simulink model "quadruped_2016"  (R2016a)
settings: Solver=ode23t  SolverMode=SingleTasking  StartTime=0.0  StopTime=8  RelTol=1e-3
values from neighbouring files (symbols this model uses):
  robot = Robot    [quadruped_sim_param.m]
undefined symbols (not defined in the file or in its folder): sigbuilder_block, X, Y, Z
undefined symbols (not defined in the file): plane
libraries: sm_lib x138, nesl_utility x66, simulink x24, Contact_Forces_Lib x12
(part 2 of 5)

== system quadruped_2016/robot/FR/hip ==
  pos : Inport
  Rigid Transform1 : sm_lib/Frames and Transforms/Rigid Transform  TranslationMethod=StandardAxis  TranslationStandardOffset=Hip.gearboxCorrection  TranslationLengthUnit=mm  TranslationStandardAxis=-Z  TranslationCartesianOffset=50  TranslationROffset=0  TranslationROffsetUnits=m  TranslationZOffset=0  TranslationZOffsetUnits=m  TranslationThetaOffset=0  TranslationThetaOffsetUnits=deg  RotationMethod=None  RotationAngleUnits=deg  RotationStandardAxis=-X  RotationAngle=180  RotationArbitraryAxis=[0 0 1]  FollAlignAxisA=+X  BaseAlignAxisA=+Y  FollAlignAxisB=+Y  BaseAlignAxisB=+Z  RotationSequenceAxes=FollowerAxes  RotationSequence=XYZ  RotationSequenceAngles=[180 0 180]  RotationSequenceAnglesUnits=deg  RotationMatrix=[1 0 0; 0 1 0; 0 0 1]
  Rigid Transform6 : sm_lib/Frames and Transforms/Rigid Transform  TranslationMethod=Cartesian  TranslationStandardOffset=0.3  TranslationLengthUnit=mm  TranslationStandardAxis=+X  TranslationCartesianOffset=Hip.legGbxOft  TranslationROffset=0  TranslationROffsetUnits=m  TranslationZOffset=0  TranslationZOffsetUnits=m  TranslationThetaOffset=0  TranslationThetaOffsetUnits=deg  RotationMethod=StandardAxis  RotationAngleUnits=deg  RotationStandardAxis=-X  RotationAngle=90  RotationArbitraryAxis=[0 0 1]  FollAlignAxisA=+X  BaseAlignAxisA=+Y  FollAlignAxisB=+Y  BaseAlignAxisB=+Z  RotationSequenceAxes=FollowerAxes  RotationSequence=XYX  RotationSequenceAngles=[0 0 0]  RotationSequenceAnglesUnits=deg  RotationMatrix=[1 0 0; 0 1 0; 0 0 1]
  Rigid Transform7 : sm_lib/Frames and Transforms/Rigid Transform  TranslationMethod=Cartesian  TranslationStandardOffset=0.3  TranslationLengthUnit=mm  TranslationStandardAxis=+X  TranslationCartesianOffset=Hip.legOft  TranslationROffset=0  TranslationROffsetUnits=m  TranslationZOffset=0  TranslationZOffsetUnits=m  TranslationThetaOffset=0  TranslationThetaOffsetUnits=deg  RotationMethod=RotationSequence  RotationAngleUnits=deg  RotationStandardAxis=-X  RotationAngle=180  RotationArbitraryAxis=[0 0 1]  FollAlignAxisA=+X  BaseAlignAxisA=+Y  FollAlignAxisB=+Y  BaseAlignAxisB=+Z  RotationSequenceAxes=FollowerAxes  RotationSequence=XYZ  RotationSequenceAngles=[0 0 180]  RotationSequenceAnglesUnits=deg  RotationMatrix=[1 0 0; 0 1 0; 0 0 1]
  Rigid Transform8 : sm_lib/Frames and Transforms/Rigid Transform  TranslationMethod=Cartesian  TranslationStandardOffset=0.3  TranslationLengthUnit=mm  TranslationStandardAxis=+X  TranslationCartesianOffset=Hip.kneeGbxOft  TranslationROffset=0  TranslationROffsetUnits=m  TranslationZOffset=0  TranslationZOffsetUnits=m  TranslationThetaOffset=0  TranslationThetaOffsetUnits=deg  RotationMethod=StandardAxis  RotationAngleUnits=deg  RotationStandardAxis=-X  RotationAngle=90  RotationArbitraryAxis=[0 0 1]  FollAlignAxisA=+X  BaseAlignAxisA=+Y  FollAlignAxisB=+Y  BaseAlignAxisB=+Z  RotationSequenceAxes=FollowerAxes  RotationSequence=XYX  RotationSequenceAngles=[0 0 0]  RotationSequenceAnglesUnits=deg  RotationMatrix=[1 0 0; 0 1 0; 0 0 1]
  Sphere to Plane Force1 : Contact_Forces_Lib/3D/Sphere to Plane Force  sphere_rad=Leg.lower_joint.sphere_rad  plane_lenx=plane_dim(1)  plane_leny=plane_dim(2)  plane_depth=plane_dim(3)/2  force_law=Linear  k_contact=1e4  b_contact=1e2  pen_full_damp_F=1e-4  pen_exponent=1  custom_param_1=1  custom_param_2=1  friction_law=Stick-Slip Continuous  mu_kinetic=Leg.lower_joint.kine_frict  mu_static=Leg.lower_joint.stat_frict  v_thr=0.001  vis_on=off  vis_opc_en=0  vis_len_plaBz=0.005  vis_clr=[0.9 0.2 0.2]  vis_opc=0.7
  Terminator : Terminator
  hip motor : sm_lib/Body Elements/Solid  GraphicAmbientColor=[0.15 0.15 0.15 1.0]  BasedOnType=Mass  CenterOfMass=[0 0 0]  CenterOfMassUnits=m  GraphicDiffuseColor=Hip.GbxColor  CylinderLength=Hip.gearboxThickness  CylinderLengthUnits=mm  CylinderRadius=Hip.gearboxRadius  CylinderRadiusUnits=mm  Density=1000  DensityUnits=kg/m^3  DoExposeReferenceFrame=on  GraphicEmissiveColor=[0.0 0.0 0.0 1.0]  ExportEntireGeometry=off  SerializedFrames=<Frames/>  MarkerShape=Sphere  MarkerSize=10  GraphicType=FromGeometry  InertiaType=CalculateFromGeometry  Mass=Hip.gearboxMass  MassUnits=g  MomentsOfInertia=[1 1 1]  MomentsOfInertiaUnits=kg*m^2  GraphicOpacity=1.0  ProductsOfInertia=[0 0 0]  ProductsOfInertiaUnits=kg*m^2  GraphicShininess=75  GraphicSpecularColor=[0.5 0.5 0.5 1.0]  GraphicVisPropType=SimpleVisualProperties  GeometryShape=Cylinder
  joint : Subsystem  mask{Joint=Hip.joint}
  knee motor : sm_lib/Body Elements/Solid  GraphicAmbientColor=[0.15 0.15 0.15 1.0]  BasedOnType=Mass  CenterOfMass=[0 0 0]  CenterOfMassUnits=m  GraphicDiffuseColor=Hip.GbxColor  CylinderLength=Hip.gearboxThickness  CylinderLengthUnits=mm  CylinderRadius=Hip.gearboxRadius  CylinderRadiusUnits=mm  Density=1000  DensityUnits=kg/m^3  DoExposeReferenceFrame=on  GraphicEmissiveColor=[0.0 0.0 0.0 1.0]  ExportEntireGeometry=off  SerializedFrames=<Frames/>  MarkerShape=Sphere  MarkerSize=10  GraphicType=FromGeometry  InertiaType=CalculateFromGeometry  Mass=Hip.gearboxMass  MassUnits=g  MomentsOfInertia=[1 1 1]  MomentsOfInertiaUnits=kg*m^2  GraphicOpacity=1.0  ProductsOfInertia=[0 0 0]  ProductsOfInertiaUnits=kg*m^2  GraphicShininess=75  GraphicSpecularColor=[0.5 0.5 0.5 1.0]  GraphicVisPropType=SimpleVisualProperties  GeometryShape=Cylinder
  leg motor : sm_lib/Body Elements/Solid  GraphicAmbientColor=[0.15 0.15 0.15 1.0]  BasedOnType=Mass  CenterOfMass=[0 0 0]  CenterOfMassUnits=m  GraphicDiffuseColor=Hip.GbxColor  CylinderLength=Hip.gearboxThickness  CylinderLengthUnits=mm  CylinderRadius=Hip.gearboxRadius  CylinderRadiusUnits=mm  Density=1000  DensityUnits=kg/m^3  DoExposeReferenceFrame=on  GraphicEmissiveColor=[0.0 0.0 0.0 1.0]  ExportEntireGeometry=off  SerializedFrames=<Frames/>  MarkerShape=Sphere  MarkerSize=10  GraphicType=FromGeometry  InertiaType=CalculateFromGeometry  Mass=Hip.gearboxMass  MassUnits=g  MomentsOfInertia=[1 1 1]  MomentsOfInertiaUnits=kg*m^2  GraphicOpacity=1.0  ProductsOfInertia=[0 0 0]  ProductsOfInertiaUnits=kg*m^2  GraphicShininess=75  GraphicSpecularColor=[0.5 0.5 0.5 1.0]  GraphicVisPropType=SimpleVisualProperties  GeometryShape=Cylinder
  B : PMIOPort  Side=Left
  F : PMIOPort  Port=2  Side=Right
  plane : PMIOPort  Port=3  Side=Right
  p : Outport
  wires:
  Sphere to Plane Force1/1 -> Terminator/1
  pos/1 -> joint/1(in)
  joint/1(p) -> p/1
  connections:
  Rigid Transform7/RConn1 -- F/RConn1
  Rigid Transform6/RConn1 -- leg motor/RConn1 -- Rigid Transform7/LConn1
  Rigid Transform8/RConn1 -- knee motor/RConn1 -- Sphere to Plane Force1/LConn1
  Sphere to Plane Force1/RConn1 -- plane/RConn1
  B/RConn1 -- Rigid Transform1/LConn1
  joint/RConn1 -- Rigid Transform6/LConn1 -- Rigid Transform8/LConn1 -- hip motor/RConn1
  Rigid Transform1/RConn1 -- joint/LConn1

== system quadruped_2016/robot/FR/leg ==
  up pos : Inport
  lo pos : Inport  Port=2
  Bus Creator : BusCreator  Inputs=2
  Sphere to Plane Force1 : Contact_Forces_Lib/3D/Sphere to Plane Force  sphere_rad=Leg.lower_joint.sphere_rad  plane_lenx=plane_dim(1)  plane_leny=plane_dim(2)  plane_depth=plane_dim(3)/2  force_law=Linear  k_contact=1e4  b_contact=1e2  pen_full_damp_F=1e-4  pen_exponent=1  custom_param_1=1  custom_param_2=1  friction_law=Stick-Slip Continuous  mu_kinetic=Leg.lower_joint.kine_frict  mu_static=Leg.lower_joint.stat_frict  v_thr=0.001  vis_on=off  vis_opc_en=0  vis_len_plaBz=0.005  vis_clr=[0.9 0.2 0.2]  vis_opc=0.7
  Sphere to Plane Force2 : Contact_Forces_Lib/3D/Sphere to Plane Force  sphere_rad=Leg.lower_joint.sphere_rad  plane_lenx=plane_dim(1)  plane_leny=plane_dim(2)  plane_depth=plane_dim(3)/2  force_law=Linear  k_contact=1e4  b_contact=1e2  pen_full_damp_F=1e-4  pen_exponent=1  custom_param_1=1  custom_param_2=1  friction_law=Stick-Slip Continuous  mu_kinetic=Leg.lower_joint.kine_frict  mu_static=Leg.lower_joint.stat_frict  v_thr=0.001  vis_on=off  vis_opc_en=0  vis_len_plaBz=0.005  vis_clr=[0.9 0.2 0.2]  vis_opc=0.7
  Terminator : Terminator
  Terminator1 : Terminator
  Top2 : sm_lib/Frames and Transforms/Rigid Transform  TranslationMethod=StandardAxis  TranslationStandardOffset=Leg.lower_joint.sphere_rad  TranslationLengthUnit=m  TranslationStandardAxis=+X  TranslationCartesianOffset=[0 0 0.1]  TranslationROffset=0  TranslationROffsetUnits=m  TranslationZOffset=0  TranslationZOffsetUnits=m  TranslationThetaOffset=0  TranslationThetaOffsetUnits=deg  RotationMethod=None  RotationAngleUnits=deg  RotationStandardAxis=+Y  RotationAngle=90  RotationArbitraryAxis=[0 0 1]  FollAlignAxisA=+X  BaseAlignAxisA=+Y  FollAlignAxisB=+Y  BaseAlignAxisB=+Z  RotationSequenceAxes=FollowerAxes  RotationSequence=XYX  RotationSequenceAngles=[0 0 0]  RotationSequenceAnglesUnits=deg  RotationMatrix=[1 0 0; 0 1 0; 0 0 1]
  lower joint : Subsystem  mask{Leg_joint=Leg.lower_joint}
  upper joint : Subsystem  mask{Leg_joint=Leg.upper_joint}
  B : PMIOPort  Side=Left
  plane : PMIOPort  Port=2  Side=Right
  p : Outport
  wires:
  Sphere to Plane Force2/1 -> Terminator/1
  Sphere to Plane Force1/1 -> Terminator1/1
  up pos/1 -> upper joint/1(pos)
  lo pos/1 -> lower joint/1(pos)
  Bus Creator/1 -> p/1
  lower joint/1(p) -> Bus Creator/1  "lower joint data"
  upper joint/1(p) -> Bus Creator/2  "upper jount data"
  connections:
  Sphere to Plane Force2/LConn1 -- upper joint/RConn1 -- lower joint/LConn1
  upper joint/LConn1 -- B/RConn1
  Top2/LConn1 -- Sphere to Plane Force1/LConn1
  plane/RConn1 -- Sphere to Plane Force1/RConn1 -- Sphere to Plane Force2/RConn1
  lower joint/RConn1 -- Top2/RConn1

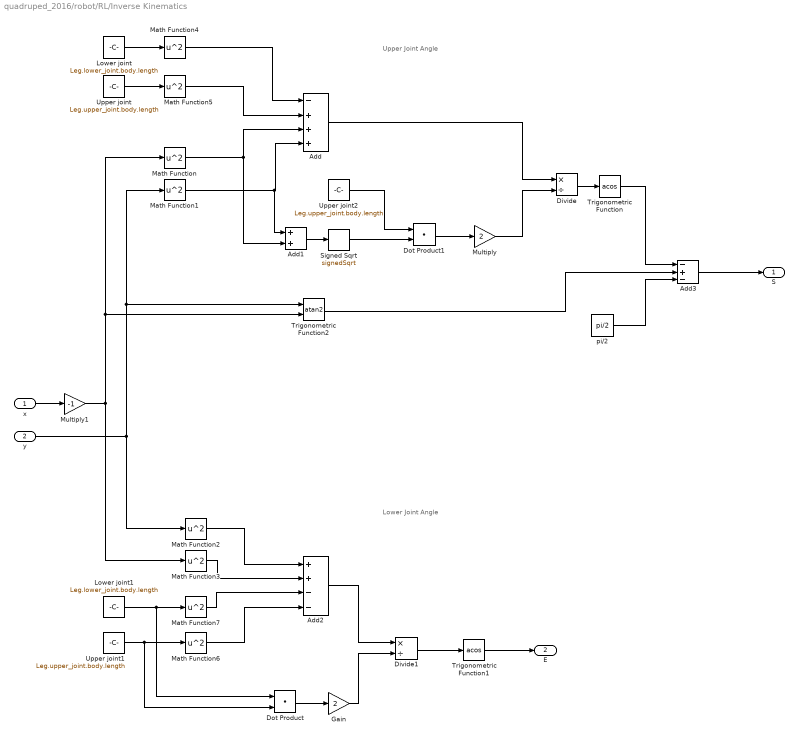
== system quadruped_2016/robot/RL/Inverse Kinematics  ==
  note: Upper Joint Angle
  note: Lower Joint Angle
  x : Inport
  y : Inport  Port=2
  Add : Sum  Inputs=-+++
  Add1 : Sum
  Add2 : Sum  Inputs=++--
  Add3 : Sum  Inputs=-+-
  Divide : Product  Inputs=*/
  Divide1 : Product  Inputs=*/
  Dot Product : DotProduct  InputSameDT=on  OutDataTypeStr=Inherit: Inherit via internal rule
  Dot Product1 : DotProduct  InputSameDT=on  OutDataTypeStr=Inherit: Inherit via internal rule
  Gain : Gain  Gain=2
  Lower joint : Constant  Value=Leg.lower_joint.body.length
  Lower joint1 : Constant  Value=Leg.lower_joint.body.length
  Math Function{,1..7} (8 alike) : Math  Operator=square  SaturateOnIntegerOverflow=on
  Multiply : Gain  Gain=2
  Multiply1 : Gain  Gain=-1
  Signed Sqrt : Sqrt  Operator=signedSqrt  SaturateOnIntegerOverflow=on
  Trigonometric Function : Trigonometry  Operator=acos
  Trigonometric Function1 : Trigonometry  Operator=acos
  Trigonometric Function2 : Trigonometry  Operator=atan2
  Upper joint : Constant  Value=Leg.upper_joint.body.length
  Upper joint1 : Constant  Value=Leg.upper_joint.body.length
  Upper joint2 : Constant  Value=Leg.upper_joint.body.length
  pi/2 : Constant  Value=pi/2
  S : Outport
  E : Outport  Port=2
  wires:
  y/1 -> Trigonometric Function2/1, Math Function1/1, Math Function2/1
  Lower joint/1 -> Math Function4/1
  Upper joint/1 -> Math Function5/1
  Math Function/1 -> Add1/2, Add/3
  Math Function1/1 -> Add1/1, Add/4
  Add1/1 -> Signed Sqrt/1
  Add/1 -> Divide/1
  Divide1/1 -> Trigonometric Function1/1
  Dot Product/1 -> Gain/1
  Add2/1 -> Divide1/1
  Gain/1 -> Divide1/2
  Divide/1 -> Trigonometric Function/1
  Trigonometric Function1/1 -> E/1
  Math Function2/1 -> Add2/1
  Math Function3/1 -> Add2/2
  Lower joint1/1 -> Math Function7/1, Dot Product/1
  Upper joint1/1 -> Dot Product/2, Math Function6/1
  Trigonometric Function/1 -> Add3/1
  Trigonometric Function2/1 -> Add3/2
  Add3/1 -> S/1
  Math Function5/1 -> Add/2
  Math Function4/1 -> Add/1
  Math Function7/1 -> Add2/3
  Math Function6/1 -> Add2/4
  Multiply/1 -> Divide/2
  Dot Product1/1 -> Multiply/1
  Signed Sqrt/1 -> Dot Product1/2
  Upper joint2/1 -> Dot Product1/1
  pi/2/1 -> Add3/3
  x/1 -> Multiply1/1
  Multiply1/1 -> Trigonometric Function2/2, Math Function/1, Math Function3/1

== system quadruped_2016/robot/RL/hip ==
  pos : Inport
  Rigid Transform1 : sm_lib/Frames and Transforms/Rigid Transform  TranslationMethod=StandardAxis  TranslationStandardOffset=Hip.gearboxCorrection  TranslationLengthUnit=mm  TranslationStandardAxis=-Z  TranslationCartesianOffset=50  TranslationROffset=0  TranslationROffsetUnits=m  TranslationZOffset=0  TranslationZOffsetUnits=m  TranslationThetaOffset=0  TranslationThetaOffsetUnits=deg  RotationMethod=None  RotationAngleUnits=deg  RotationStandardAxis=-X  RotationAngle=180  RotationArbitraryAxis=[0 0 1]  FollAlignAxisA=+X  BaseAlignAxisA=+Y  FollAlignAxisB=+Y  BaseAlignAxisB=+Z  RotationSequenceAxes=FollowerAxes  RotationSequence=XYZ  RotationSequenceAngles=[180 0 180]  RotationSequenceAnglesUnits=deg  RotationMatrix=[1 0 0; 0 1 0; 0 0 1]
  Rigid Transform6 : sm_lib/Frames and Transforms/Rigid Transform  TranslationMethod=Cartesian  TranslationStandardOffset=0.3  TranslationLengthUnit=mm  TranslationStandardAxis=+X  TranslationCartesianOffset=Hip.legGbxOft  TranslationROffset=0  TranslationROffsetUnits=m  TranslationZOffset=0  TranslationZOffsetUnits=m  TranslationThetaOffset=0  TranslationThetaOffsetUnits=deg  RotationMethod=StandardAxis  RotationAngleUnits=deg  RotationStandardAxis=-X  RotationAngle=90  RotationArbitraryAxis=[0 0 1]  FollAlignAxisA=+X  BaseAlignAxisA=+Y  FollAlignAxisB=+Y  BaseAlignAxisB=+Z  RotationSequenceAxes=FollowerAxes  RotationSequence=XYX  RotationSequenceAngles=[0 0 0]  RotationSequenceAnglesUnits=deg  RotationMatrix=[1 0 0; 0 1 0; 0 0 1]
  Rigid Transform7 : sm_lib/Frames and Transforms/Rigid Transform  TranslationMethod=Cartesian  TranslationStandardOffset=0.3  TranslationLengthUnit=mm  TranslationStandardAxis=+X  TranslationCartesianOffset=Hip.legOft  TranslationROffset=0  TranslationROffsetUnits=m  TranslationZOffset=0  TranslationZOffsetUnits=m  TranslationThetaOffset=0  TranslationThetaOffsetUnits=deg  RotationMethod=RotationSequence  RotationAngleUnits=deg  RotationStandardAxis=-X  RotationAngle=180  RotationArbitraryAxis=[0 0 1]  FollAlignAxisA=+X  BaseAlignAxisA=+Y  FollAlignAxisB=+Y  BaseAlignAxisB=+Z  RotationSequenceAxes=FollowerAxes  RotationSequence=XYZ  RotationSequenceAngles=[0 0 180]  RotationSequenceAnglesUnits=deg  RotationMatrix=[1 0 0; 0 1 0; 0 0 1]
  Rigid Transform8 : sm_lib/Frames and Transforms/Rigid Transform  TranslationMethod=Cartesian  TranslationStandardOffset=0.3  TranslationLengthUnit=mm  TranslationStandardAxis=+X  TranslationCartesianOffset=Hip.kneeGbxOft  TranslationROffset=0  TranslationROffsetUnits=m  TranslationZOffset=0  TranslationZOffsetUnits=m  TranslationThetaOffset=0  TranslationThetaOffsetUnits=deg  RotationMethod=StandardAxis  RotationAngleUnits=deg  RotationStandardAxis=-X  RotationAngle=90  RotationArbitraryAxis=[0 0 1]  FollAlignAxisA=+X  BaseAlignAxisA=+Y  FollAlignAxisB=+Y  BaseAlignAxisB=+Z  RotationSequenceAxes=FollowerAxes  RotationSequence=XYX  RotationSequenceAngles=[0 0 0]  RotationSequenceAnglesUnits=deg  RotationMatrix=[1 0 0; 0 1 0; 0 0 1]
  Sphere to Plane Force1 : Contact_Forces_Lib/3D/Sphere to Plane Force  sphere_rad=Leg.lower_joint.sphere_rad  plane_lenx=plane_dim(1)  plane_leny=plane_dim(2)  plane_depth=plane_dim(3)/2  force_law=Linear  k_contact=1e4  b_contact=1e2  pen_full_damp_F=1e-4  pen_exponent=1  custom_param_1=1  custom_param_2=1  friction_law=Stick-Slip Continuous  mu_kinetic=Leg.lower_joint.kine_frict  mu_static=Leg.lower_joint.stat_frict  v_thr=0.001  vis_on=off  vis_opc_en=0  vis_len_plaBz=0.005  vis_clr=[0.9 0.2 0.2]  vis_opc=0.7
  Terminator : Terminator
  hip motor : sm_lib/Body Elements/Solid  GraphicAmbientColor=[0.15 0.15 0.15 1.0]  BasedOnType=Mass  CenterOfMass=[0 0 0]  CenterOfMassUnits=m  GraphicDiffuseColor=Hip.GbxColor  CylinderLength=Hip.gearboxThickness  CylinderLengthUnits=mm  CylinderRadius=Hip.gearboxRadius  CylinderRadiusUnits=mm  Density=1000  DensityUnits=kg/m^3  DoExposeReferenceFrame=on  GraphicEmissiveColor=[0.0 0.0 0.0 1.0]  ExportEntireGeometry=off  SerializedFrames=<Frames/>  MarkerShape=Sphere  MarkerSize=10  GraphicType=FromGeometry  InertiaType=CalculateFromGeometry  Mass=Hip.gearboxMass  MassUnits=g  MomentsOfInertia=[1 1 1]  MomentsOfInertiaUnits=kg*m^2  GraphicOpacity=1.0  ProductsOfInertia=[0 0 0]  ProductsOfInertiaUnits=kg*m^2  GraphicShininess=75  GraphicSpecularColor=[0.5 0.5 0.5 1.0]  GraphicVisPropType=SimpleVisualProperties  GeometryShape=Cylinder
  joint : Subsystem  mask{Joint=Hip.joint}
  knee motor : sm_lib/Body Elements/Solid  GraphicAmbientColor=[0.15 0.15 0.15 1.0]  BasedOnType=Mass  CenterOfMass=[0 0 0]  CenterOfMassUnits=m  GraphicDiffuseColor=Hip.GbxColor  CylinderLength=Hip.gearboxThickness  CylinderLengthUnits=mm  CylinderRadius=Hip.gearboxRadius  CylinderRadiusUnits=mm  Density=1000  DensityUnits=kg/m^3  DoExposeReferenceFrame=on  GraphicEmissiveColor=[0.0 0.0 0.0 1.0]  ExportEntireGeometry=off  SerializedFrames=<Frames/>  MarkerShape=Sphere  MarkerSize=10  GraphicType=FromGeometry  InertiaType=CalculateFromGeometry  Mass=Hip.gearboxMass  MassUnits=g  MomentsOfInertia=[1 1 1]  MomentsOfInertiaUnits=kg*m^2  GraphicOpacity=1.0  ProductsOfInertia=[0 0 0]  ProductsOfInertiaUnits=kg*m^2  GraphicShininess=75  GraphicSpecularColor=[0.5 0.5 0.5 1.0]  GraphicVisPropType=SimpleVisualProperties  GeometryShape=Cylinder
  leg motor : sm_lib/Body Elements/Solid  GraphicAmbientColor=[0.15 0.15 0.15 1.0]  BasedOnType=Mass  CenterOfMass=[0 0 0]  CenterOfMassUnits=m  GraphicDiffuseColor=Hip.GbxColor  CylinderLength=Hip.gearboxThickness  CylinderLengthUnits=mm  CylinderRadius=Hip.gearboxRadius  CylinderRadiusUnits=mm  Density=1000  DensityUnits=kg/m^3  DoExposeReferenceFrame=on  GraphicEmissiveColor=[0.0 0.0 0.0 1.0]  ExportEntireGeometry=off  SerializedFrames=<Frames/>  MarkerShape=Sphere  MarkerSize=10  GraphicType=FromGeometry  InertiaType=CalculateFromGeometry  Mass=Hip.gearboxMass  MassUnits=g  MomentsOfInertia=[1 1 1]  MomentsOfInertiaUnits=kg*m^2  GraphicOpacity=1.0  ProductsOfInertia=[0 0 0]  ProductsOfInertiaUnits=kg*m^2  GraphicShininess=75  GraphicSpecularColor=[0.5 0.5 0.5 1.0]  GraphicVisPropType=SimpleVisualProperties  GeometryShape=Cylinder
  B : PMIOPort  Side=Left
  F : PMIOPort  Port=2  Side=Right
  plane : PMIOPort  Port=3  Side=Right
  p : Outport
  wires:
  Sphere to Plane Force1/1 -> Terminator/1
  pos/1 -> joint/1(in)
  joint/1(p) -> p/1
  connections:
  Rigid Transform7/RConn1 -- F/RConn1
  Rigid Transform6/RConn1 -- leg motor/RConn1 -- Rigid Transform7/LConn1
  Rigid Transform8/RConn1 -- knee motor/RConn1 -- Sphere to Plane Force1/LConn1
  Sphere to Plane Force1/RConn1 -- plane/RConn1
  B/RConn1 -- Rigid Transform1/LConn1
  joint/RConn1 -- Rigid Transform6/LConn1 -- Rigid Transform8/LConn1 -- hip motor/RConn1
  Rigid Transform1/RConn1 -- joint/LConn1

== system quadruped_2016/robot/RL/leg ==
  up pos : Inport
  lo pos : Inport  Port=2
  Bus Creator : BusCreator  Inputs=2
  Sphere to Plane Force1 : Contact_Forces_Lib/3D/Sphere to Plane Force  sphere_rad=Leg.lower_joint.sphere_rad  plane_lenx=plane_dim(1)  plane_leny=plane_dim(2)  plane_depth=plane_dim(3)/2  force_law=Linear  k_contact=1e4  b_contact=1e2  pen_full_damp_F=1e-4  pen_exponent=1  custom_param_1=1  custom_param_2=1  friction_law=Stick-Slip Continuous  mu_kinetic=Leg.lower_joint.kine_frict  mu_static=Leg.lower_joint.stat_frict  v_thr=0.001  vis_on=off  vis_opc_en=0  vis_len_plaBz=0.005  vis_clr=[0.9 0.2 0.2]  vis_opc=0.7
  Sphere to Plane Force2 : Contact_Forces_Lib/3D/Sphere to Plane Force  sphere_rad=Leg.lower_joint.sphere_rad  plane_lenx=plane_dim(1)  plane_leny=plane_dim(2)  plane_depth=plane_dim(3)/2  force_law=Linear  k_contact=1e4  b_contact=1e2  pen_full_damp_F=1e-4  pen_exponent=1  custom_param_1=1  custom_param_2=1  friction_law=Stick-Slip Continuous  mu_kinetic=Leg.lower_joint.kine_frict  mu_static=Leg.lower_joint.stat_frict  v_thr=0.001  vis_on=off  vis_opc_en=0  vis_len_plaBz=0.005  vis_clr=[0.9 0.2 0.2]  vis_opc=0.7
  Terminator : Terminator
  Terminator1 : Terminator
  Top2 : sm_lib/Frames and Transforms/Rigid Transform  TranslationMethod=StandardAxis  TranslationStandardOffset=Leg.lower_joint.sphere_rad  TranslationLengthUnit=m  TranslationStandardAxis=+X  TranslationCartesianOffset=[0 0 0.1]  TranslationROffset=0  TranslationROffsetUnits=m  TranslationZOffset=0  TranslationZOffsetUnits=m  TranslationThetaOffset=0  TranslationThetaOffsetUnits=deg  RotationMethod=None  RotationAngleUnits=deg  RotationStandardAxis=+Y  RotationAngle=90  RotationArbitraryAxis=[0 0 1]  FollAlignAxisA=+X  BaseAlignAxisA=+Y  FollAlignAxisB=+Y  BaseAlignAxisB=+Z  RotationSequenceAxes=FollowerAxes  RotationSequence=XYX  RotationSequenceAngles=[0 0 0]  RotationSequenceAnglesUnits=deg  RotationMatrix=[1 0 0; 0 1 0; 0 0 1]
  lower joint : Subsystem  mask{Leg_joint=Leg.lower_joint}
  upper joint : Subsystem  mask{Leg_joint=Leg.upper_joint}
  B : PMIOPort  Side=Left
  plane : PMIOPort  Port=2  Side=Right
  p : Outport
  wires:
  Sphere to Plane Force2/1 -> Terminator/1
  Sphere to Plane Force1/1 -> Terminator1/1
  up pos/1 -> upper joint/1(pos)
  lo pos/1 -> lower joint/1(pos)
  Bus Creator/1 -> p/1
  lower joint/1(p) -> Bus Creator/1  "lower joint data"
  upper joint/1(p) -> Bus Creator/2  "upper jount data"
  connections:
  Sphere to Plane Force2/LConn1 -- upper joint/RConn1 -- lower joint/LConn1
  upper joint/LConn1 -- B/RConn1
  Top2/LConn1 -- Sphere to Plane Force1/LConn1
  plane/RConn1 -- Sphere to Plane Force1/RConn1 -- Sphere to Plane Force2/RConn1
  lower joint/RConn1 -- Top2/RConn1

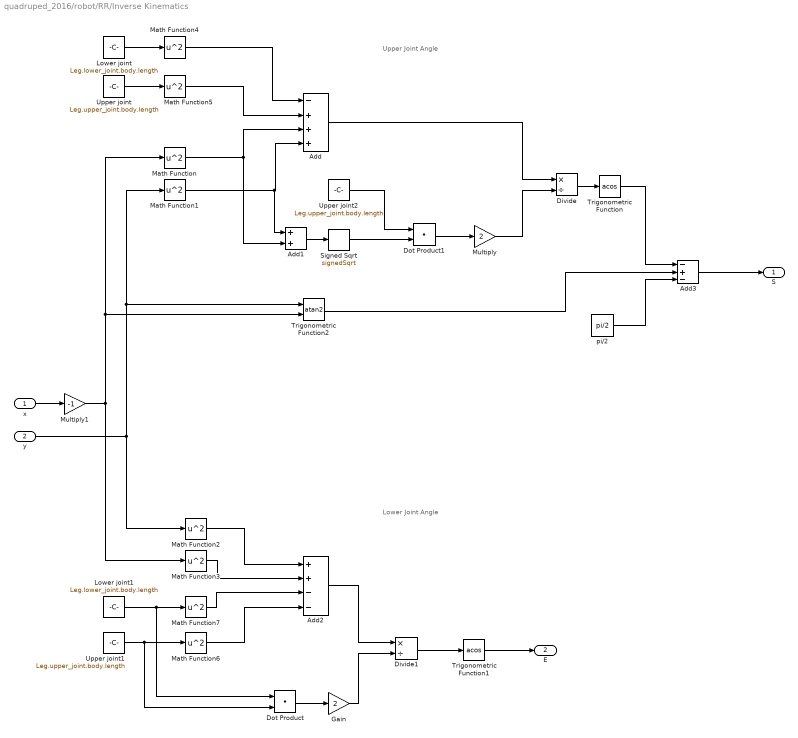
== system quadruped_2016/robot/RR/Inverse Kinematics  ==
  note: Upper Joint Angle
  note: Lower Joint Angle
  x : Inport
  y : Inport  Port=2
  Add : Sum  Inputs=-+++
  Add1 : Sum
  Add2 : Sum  Inputs=++--
  Add3 : Sum  Inputs=-+-
  Divide : Product  Inputs=*/
  Divide1 : Product  Inputs=*/
  Dot Product : DotProduct  InputSameDT=on  OutDataTypeStr=Inherit: Inherit via internal rule
  Dot Product1 : DotProduct  InputSameDT=on  OutDataTypeStr=Inherit: Inherit via internal rule
  Gain : Gain  Gain=2
  Lower joint : Constant  Value=Leg.lower_joint.body.length
  Lower joint1 : Constant  Value=Leg.lower_joint.body.length
  Math Function{,1..7} (8 alike) : Math  Operator=square  SaturateOnIntegerOverflow=on
  Multiply : Gain  Gain=2
  Multiply1 : Gain  Gain=-1
  Signed Sqrt : Sqrt  Operator=signedSqrt  SaturateOnIntegerOverflow=on
  Trigonometric Function : Trigonometry  Operator=acos
  Trigonometric Function1 : Trigonometry  Operator=acos
  Trigonometric Function2 : Trigonometry  Operator=atan2
  Upper joint : Constant  Value=Leg.upper_joint.body.length
  Upper joint1 : Constant  Value=Leg.upper_joint.body.length
  Upper joint2 : Constant  Value=Leg.upper_joint.body.length
  pi/2 : Constant  Value=pi/2
  S : Outport
  E : Outport  Port=2
  wires:
  y/1 -> Trigonometric Function2/1, Math Function1/1, Math Function2/1
  Lower joint/1 -> Math Function4/1
  Upper joint/1 -> Math Function5/1
  Math Function/1 -> Add1/2, Add/3
  Math Function1/1 -> Add1/1, Add/4
  Add1/1 -> Signed Sqrt/1
  Add/1 -> Divide/1
  Divide1/1 -> Trigonometric Function1/1
  Dot Product/1 -> Gain/1
  Add2/1 -> Divide1/1
  Gain/1 -> Divide1/2
  Divide/1 -> Trigonometric Function/1
  Trigonometric Function1/1 -> E/1
  Math Function2/1 -> Add2/1
  Math Function3/1 -> Add2/2
  Lower joint1/1 -> Math Function7/1, Dot Product/1
  Upper joint1/1 -> Dot Product/2, Math Function6/1
  Trigonometric Function/1 -> Add3/1
  Trigonometric Function2/1 -> Add3/2
  Add3/1 -> S/1
  Math Function5/1 -> Add/2
  Math Function4/1 -> Add/1
  Math Function7/1 -> Add2/3
  Math Function6/1 -> Add2/4
  Multiply/1 -> Divide/2
  Dot Product1/1 -> Multiply/1
  Signed Sqrt/1 -> Dot Product1/2
  Upper joint2/1 -> Dot Product1/1
  pi/2/1 -> Add3/3
  x/1 -> Multiply1/1
  Multiply1/1 -> Trigonometric Function2/2, Math Function/1, Math Function3/1

== system quadruped_2016/robot/RR/hip ==
  pos : Inport
  Rigid Transform1 : sm_lib/Frames and Transforms/Rigid Transform  TranslationMethod=StandardAxis  TranslationStandardOffset=Hip.gearboxCorrection  TranslationLengthUnit=mm  TranslationStandardAxis=-Z  TranslationCartesianOffset=50  TranslationROffset=0  TranslationROffsetUnits=m  TranslationZOffset=0  TranslationZOffsetUnits=m  TranslationThetaOffset=0  TranslationThetaOffsetUnits=deg  RotationMethod=None  RotationAngleUnits=deg  RotationStandardAxis=-X  RotationAngle=180  RotationArbitraryAxis=[0 0 1]  FollAlignAxisA=+X  BaseAlignAxisA=+Y  FollAlignAxisB=+Y  BaseAlignAxisB=+Z  RotationSequenceAxes=FollowerAxes  RotationSequence=XYZ  RotationSequenceAngles=[180 0 180]  RotationSequenceAnglesUnits=deg  RotationMatrix=[1 0 0; 0 1 0; 0 0 1]
  Rigid Transform6 : sm_lib/Frames and Transforms/Rigid Transform  TranslationMethod=Cartesian  TranslationStandardOffset=0.3  TranslationLengthUnit=mm  TranslationStandardAxis=+X  TranslationCartesianOffset=Hip.legGbxOft  TranslationROffset=0  TranslationROffsetUnits=m  TranslationZOffset=0  TranslationZOffsetUnits=m  TranslationThetaOffset=0  TranslationThetaOffsetUnits=deg  RotationMethod=StandardAxis  RotationAngleUnits=deg  RotationStandardAxis=-X  RotationAngle=90  RotationArbitraryAxis=[0 0 1]  FollAlignAxisA=+X  BaseAlignAxisA=+Y  FollAlignAxisB=+Y  BaseAlignAxisB=+Z  RotationSequenceAxes=FollowerAxes  RotationSequence=XYX  RotationSequenceAngles=[0 0 0]  RotationSequenceAnglesUnits=deg  RotationMatrix=[1 0 0; 0 1 0; 0 0 1]
  Rigid Transform7 : sm_lib/Frames and Transforms/Rigid Transform  TranslationMethod=Cartesian  TranslationStandardOffset=0.3  TranslationLengthUnit=mm  TranslationStandardAxis=+X  TranslationCartesianOffset=Hip.legOft  TranslationROffset=0  TranslationROffsetUnits=m  TranslationZOffset=0  TranslationZOffsetUnits=m  TranslationThetaOffset=0  TranslationThetaOffsetUnits=deg  RotationMethod=RotationSequence  RotationAngleUnits=deg  RotationStandardAxis=-X  RotationAngle=180  RotationArbitraryAxis=[0 0 1]  FollAlignAxisA=+X  BaseAlignAxisA=+Y  FollAlignAxisB=+Y  BaseAlignAxisB=+Z  RotationSequenceAxes=FollowerAxes  RotationSequence=XYZ  RotationSequenceAngles=[0 0 180]  RotationSequenceAnglesUnits=deg  RotationMatrix=[1 0 0; 0 1 0; 0 0 1]
  Rigid Transform8 : sm_lib/Frames and Transforms/Rigid Transform  TranslationMethod=Cartesian  TranslationStandardOffset=0.3  TranslationLengthUnit=mm  TranslationStandardAxis=+X  TranslationCartesianOffset=Hip.kneeGbxOft  TranslationROffset=0  TranslationROffsetUnits=m  TranslationZOffset=0  TranslationZOffsetUnits=m  TranslationThetaOffset=0  TranslationThetaOffsetUnits=deg  RotationMethod=StandardAxis  RotationAngleUnits=deg  RotationStandardAxis=-X  RotationAngle=90  RotationArbitraryAxis=[0 0 1]  FollAlignAxisA=+X  BaseAlignAxisA=+Y  FollAlignAxisB=+Y  BaseAlignAxisB=+Z  RotationSequenceAxes=FollowerAxes  RotationSequence=XYX  RotationSequenceAngles=[0 0 0]  RotationSequenceAnglesUnits=deg  RotationMatrix=[1 0 0; 0 1 0; 0 0 1]
  Sphere to Plane Force1 : Contact_Forces_Lib/3D/Sphere to Plane Force  sphere_rad=Leg.lower_joint.sphere_rad  plane_lenx=plane_dim(1)  plane_leny=plane_dim(2)  plane_depth=plane_dim(3)/2  force_law=Linear  k_contact=1e4  b_contact=1e2  pen_full_damp_F=1e-4  pen_exponent=1  custom_param_1=1  custom_param_2=1  friction_law=Stick-Slip Continuous  mu_kinetic=Leg.lower_joint.kine_frict  mu_static=Leg.lower_joint.stat_frict  v_thr=0.001  vis_on=off  vis_opc_en=0  vis_len_plaBz=0.005  vis_clr=[0.9 0.2 0.2]  vis_opc=0.7
  Terminator : Terminator
  hip motor : sm_lib/Body Elements/Solid  GraphicAmbientColor=[0.15 0.15 0.15 1.0]  BasedOnType=Mass  CenterOfMass=[0 0 0]  CenterOfMassUnits=m  GraphicDiffuseColor=Hip.GbxColor  CylinderLength=Hip.gearboxThickness  CylinderLengthUnits=mm  CylinderRadius=Hip.gearboxRadius  CylinderRadiusUnits=mm  Density=1000  DensityUnits=kg/m^3  DoExposeReferenceFrame=on  GraphicEmissiveColor=[0.0 0.0 0.0 1.0]  ExportEntireGeometry=off  SerializedFrames=<Frames/>  MarkerShape=Sphere  MarkerSize=10  GraphicType=FromGeometry  InertiaType=CalculateFromGeometry  Mass=Hip.gearboxMass  MassUnits=g  MomentsOfInertia=[1 1 1]  MomentsOfInertiaUnits=kg*m^2  GraphicOpacity=1.0  ProductsOfInertia=[0 0 0]  ProductsOfInertiaUnits=kg*m^2  GraphicShininess=75  GraphicSpecularColor=[0.5 0.5 0.5 1.0]  GraphicVisPropType=SimpleVisualProperties  GeometryShape=Cylinder
  joint : Subsystem  mask{Joint=Hip.joint}
  knee motor : sm_lib/Body Elements/Solid  GraphicAmbientColor=[0.15 0.15 0.15 1.0]  BasedOnType=Mass  CenterOfMass=[0 0 0]  CenterOfMassUnits=m  GraphicDiffuseColor=Hip.GbxColor  CylinderLength=Hip.gearboxThickness  CylinderLengthUnits=mm  CylinderRadius=Hip.gearboxRadius  CylinderRadiusUnits=mm  Density=1000  DensityUnits=kg/m^3  DoExposeReferenceFrame=on  GraphicEmissiveColor=[0.0 0.0 0.0 1.0]  ExportEntireGeometry=off  SerializedFrames=<Frames/>  MarkerShape=Sphere  MarkerSize=10  GraphicType=FromGeometry  InertiaType=CalculateFromGeometry  Mass=Hip.gearboxMass  MassUnits=g  MomentsOfInertia=[1 1 1]  MomentsOfInertiaUnits=kg*m^2  GraphicOpacity=1.0  ProductsOfInertia=[0 0 0]  ProductsOfInertiaUnits=kg*m^2  GraphicShininess=75  GraphicSpecularColor=[0.5 0.5 0.5 1.0]  GraphicVisPropType=SimpleVisualProperties  GeometryShape=Cylinder
  leg motor : sm_lib/Body Elements/Solid  GraphicAmbientColor=[0.15 0.15 0.15 1.0]  BasedOnType=Mass  CenterOfMass=[0 0 0]  CenterOfMassUnits=m  GraphicDiffuseColor=Hip.GbxColor  CylinderLength=Hip.gearboxThickness  CylinderLengthUnits=mm  CylinderRadius=Hip.gearboxRadius  CylinderRadiusUnits=mm  Density=1000  DensityUnits=kg/m^3  DoExposeReferenceFrame=on  GraphicEmissiveColor=[0.0 0.0 0.0 1.0]  ExportEntireGeometry=off  SerializedFrames=<Frames/>  MarkerShape=Sphere  MarkerSize=10  GraphicType=FromGeometry  InertiaType=CalculateFromGeometry  Mass=Hip.gearboxMass  MassUnits=g  MomentsOfInertia=[1 1 1]  MomentsOfInertiaUnits=kg*m^2  GraphicOpacity=1.0  ProductsOfInertia=[0 0 0]  ProductsOfInertiaUnits=kg*m^2  GraphicShininess=75  GraphicSpecularColor=[0.5 0.5 0.5 1.0]  GraphicVisPropType=SimpleVisualProperties  GeometryShape=Cylinder
  B : PMIOPort  Side=Left
  F : PMIOPort  Port=2  Side=Right
  plane : PMIOPort  Port=3  Side=Right
  p : Outport
  wires:
  Sphere to Plane Force1/1 -> Terminator/1
  pos/1 -> joint/1(in)
  joint/1(p) -> p/1
  connections:
  Rigid Transform7/RConn1 -- F/RConn1
  Rigid Transform6/RConn1 -- leg motor/RConn1 -- Rigid Transform7/LConn1
  Rigid Transform8/RConn1 -- knee motor/RConn1 -- Sphere to Plane Force1/LConn1
  Sphere to Plane Force1/RConn1 -- plane/RConn1
  B/RConn1 -- Rigid Transform1/LConn1
  joint/RConn1 -- Rigid Transform6/LConn1 -- Rigid Transform8/LConn1 -- hip motor/RConn1
  Rigid Transform1/RConn1 -- joint/LConn1

== system quadruped_2016/robot/RR/leg ==
  up pos : Inport
  lo pos : Inport  Port=2
  Bus Creator : BusCreator  Inputs=2
  Sphere to Plane Force1 : Contact_Forces_Lib/3D/Sphere to Plane Force  sphere_rad=Leg.lower_joint.sphere_rad  plane_lenx=plane_dim(1)  plane_leny=plane_dim(2)  plane_depth=plane_dim(3)/2  force_law=Linear  k_contact=1e4  b_contact=1e2  pen_full_damp_F=1e-4  pen_exponent=1  custom_param_1=1  custom_param_2=1  friction_law=Stick-Slip Continuous  mu_kinetic=Leg.lower_joint.kine_frict  mu_static=Leg.lower_joint.stat_frict  v_thr=0.001  vis_on=off  vis_opc_en=0  vis_len_plaBz=0.005  vis_clr=[0.9 0.2 0.2]  vis_opc=0.7
  Sphere to Plane Force2 : Contact_Forces_Lib/3D/Sphere to Plane Force  sphere_rad=Leg.lower_joint.sphere_rad  plane_lenx=plane_dim(1)  plane_leny=plane_dim(2)  plane_depth=plane_dim(3)/2  force_law=Linear  k_contact=1e4  b_contact=1e2  pen_full_damp_F=1e-4  pen_exponent=1  custom_param_1=1  custom_param_2=1  friction_law=Stick-Slip Continuous  mu_kinetic=Leg.lower_joint.kine_frict  mu_static=Leg.lower_joint.stat_frict  v_thr=0.001  vis_on=off  vis_opc_en=0  vis_len_plaBz=0.005  vis_clr=[0.9 0.2 0.2]  vis_opc=0.7
  Terminator : Terminator
  Terminator1 : Terminator
  Top2 : sm_lib/Frames and Transforms/Rigid Transform  TranslationMethod=StandardAxis  TranslationStandardOffset=Leg.lower_joint.sphere_rad  TranslationLengthUnit=m  TranslationStandardAxis=+X  TranslationCartesianOffset=[0 0 0.1]  TranslationROffset=0  TranslationROffsetUnits=m  TranslationZOffset=0  TranslationZOffsetUnits=m  TranslationThetaOffset=0  TranslationThetaOffsetUnits=deg  RotationMethod=None  RotationAngleUnits=deg  RotationStandardAxis=+Y  RotationAngle=90  RotationArbitraryAxis=[0 0 1]  FollAlignAxisA=+X  BaseAlignAxisA=+Y  FollAlignAxisB=+Y  BaseAlignAxisB=+Z  RotationSequenceAxes=FollowerAxes  RotationSequence=XYX  RotationSequenceAngles=[0 0 0]  RotationSequenceAnglesUnits=deg  RotationMatrix=[1 0 0; 0 1 0; 0 0 1]
  lower joint : Subsystem  mask{Leg_joint=Leg.lower_joint}
  upper joint : Subsystem  mask{Leg_joint=Leg.upper_joint}
  B : PMIOPort  Side=Left
  plane : PMIOPort  Port=2  Side=Right
  p : Outport
  wires:
  Sphere to Plane Force2/1 -> Terminator/1
  Sphere to Plane Force1/1 -> Terminator1/1
  up pos/1 -> upper joint/1(pos)
  lo pos/1 -> lower joint/1(pos)
  Bus Creator/1 -> p/1
  lower joint/1(p) -> Bus Creator/1  "lower joint data"
  upper joint/1(p) -> Bus Creator/2  "upper jount data"
  connections:
  Sphere to Plane Force2/LConn1 -- upper joint/RConn1 -- lower joint/LConn1
  upper joint/LConn1 -- B/RConn1
  Top2/LConn1 -- Sphere to Plane Force1/LConn1
  plane/RConn1 -- Sphere to Plane Force1/RConn1 -- Sphere to Plane Force2/RConn1
  lower joint/RConn1 -- Top2/RConn1

== system quadruped_2016/robot/robot body/robot position ==
  Bus Creator : BusCreator  Inputs=5
  PS-Simulink Converter1 : nesl_utility/PS-Simulink Converter  PhysicalDomain=network_engine_domain  SubClassName=ps_output  LeftPortType=input  RightPortType=output  PseudoPeriodic=off  Frequencies=[]  Unit=cm  AffineConversion=off
  PS-Simulink Converter2 : nesl_utility/PS-Simulink Converter  PhysicalDomain=network_engine_domain  SubClassName=ps_output  LeftPortType=input  RightPortType=output  PseudoPeriodic=off  Frequencies=[]  Unit=inherit  AffineConversion=off
  PS-Simulink Converter3 : nesl_utility/PS-Simulink Converter  PhysicalDomain=network_engine_domain  SubClassName=ps_output  LeftPortType=input  RightPortType=output  PseudoPeriodic=off  Frequencies=[]  Unit=inherit  AffineConversion=off
  PS-Simulink Converter4 : nesl_utility/PS-Simulink Converter  PhysicalDomain=network_engine_domain  SubClassName=ps_output  LeftPortType=input  RightPortType=output  PseudoPeriodic=off  Frequencies=[]  Unit=cm  AffineConversion=off
  PS-Simulink Converter5 : nesl_utility/PS-Simulink Converter  PhysicalDomain=network_engine_domain  SubClassName=ps_output  LeftPortType=input  RightPortType=output  PseudoPeriodic=off  Frequencies=[]  Unit=cm  AffineConversion=off
  Transform Sensor : sm_lib/Frames and Transforms/Transform Sensor  MeasurementFrame=World  SenseAngle=on  SenseAxis=on  SenseAngle1=off  SenseAngle2=off  SenseAngle3=off  SenseQ=off  SenseR=off  SenseOmegaX=off  SenseOmegaY=off  SenseOmegaZ=off  SenseOmega1=off  SenseOmega2=off  SenseOmega3=off  SenseQDot=off  SenseRDot=off  SenseAlphaX=off  SenseAlphaY=off  SenseAlphaZ=off  SenseAlpha1=off  SenseAlpha2=off  SenseAlpha3=off  SenseQDDot=off  SenseRDDot=off  SenseX=on  SenseY=on  SenseZ=on  SenseRad=off  SenseAzim=off  SenseDist=off  SenseInc=off  SenseXDot=off  SenseYDot=off  SenseZDot=off  SenseRadDot=off  SenseAzimDot=off  SenseDistDot=off  SenseIncDot=off  SenseXDDot=off  SenseYDDot=off  SenseZDDot=off  SenseRadDDot=off  SenseAzimDDot=off  SenseDistDDot=off  SenseIncDDot=off
  F : PMIOPort  Side=Left
  B : PMIOPort  Port=2  Side=Right
  p : Outport
  wires:
  PS-Simulink Converter3/1 -> Bus Creator/1  "q"
  PS-Simulink Converter2/1 -> Bus Creator/2  "axs"
  PS-Simulink Converter1/1 -> Bus Creator/3  "x"
  PS-Simulink Converter4/1 -> Bus Creator/4  "y"
  PS-Simulink Converter5/1 -> Bus Creator/5  "z"
  Bus Creator/1 -> p/1
  connections:
  Transform Sensor/RConn2 -- PS-Simulink Converter3/LConn1
  Transform Sensor/RConn3 -- PS-Simulink Converter2/LConn1
  Transform Sensor/RConn4 -- PS-Simulink Converter1/LConn1
  Transform Sensor/RConn5 -- PS-Simulink Converter4/LConn1
  Transform Sensor/RConn6 -- PS-Simulink Converter5/LConn1
  Transform Sensor/LConn1 -- B/RConn1
  F/RConn1 -- Transform Sensor/RConn1

== system quadruped_2016/robot/FL/hip/joint ==
  in : Inport
  Abs1 : Abs
  Bus Creator1 : BusCreator  Inputs=4
  Bus Creator2 : BusCreator  Inputs=3
  "Hip joint " : sm_lib/Joints/Revolute Joint  JointMode=Normal  SenseConstraintForce=off  SenseConstraintForceX=off  SenseConstraintForceY=off  SenseConstraintForceZ=off  SenseConstraintTorque=off  SenseConstraintTorqueX=off  SenseConstraintTorqueY=off  SenseConstraintTorqueZ=off  SenseTotalForce=off  SenseTotalForceX=off  SenseTotalForceY=off  SenseTotalForceZ=off  SenseTotalTorque=off  SenseTotalTorqueX=off  SenseTotalTorqueY=off  SenseTotalTorqueZ=off  CompositeWrenchDir=FollowerOnBase  CompositeWrenchFrame=BaseFrame  EquilibriumPosition=0  EquilibriumPositionUnits=rad  SpringStiffness=Joint.stiffness  SpringStiffnessUnits=N*m/deg  DampingCoefficient=Joint.damping  DampingCoefficientUnits=N*m/(deg/s)  TorqueActuationMode=InputTorque  MotionActuationMode=ComputedMotion  SensePosition=on  SenseVelocity=on  SenseAcceleration=on  SenseTorqueForce=on  SenseLowerLimitTorqueForce=off  SenseUpperLimitTorqueForce=off  LowerLimitSpecify=off  LowerLimitBound=-90  LowerLimitBoundUnits=deg  LowerLimitStiffness=1e4  LowerLimitStiffnessUnits=N*m/deg  LowerLimitDamping=10  LowerLimitDampingUnits=N*m/(deg/s)  LowerLimitTransitionRegionWidth=0.1  LowerLimitTransitionRegionWidthUnits=deg  UpperLimitSpecify=off  UpperLimitBound=90  UpperLimitBoundUnits=deg  UpperLimitStiffness=1e4  UpperLimitStiffnessUnits=N*m/deg  UpperLimitDamping=10  UpperLimitDampingUnits=N*m/(deg/s)  UpperLimitTransitionRegionWidth=0.1  UpperLimitTransitionRegionWidthUnits=deg  PositionTargetSpecify=on  PositionTargetPriority=High  PositionTargetValue=Joint.base_angle  PositionTargetValueUnits=deg  VelocityTargetSpecify=off  VelocityTargetPriority=High  VelocityTargetValue=0  VelocityTargetValueUnits=deg/s
  PS-Simulink Converter3 : nesl_utility/PS-Simulink Converter  PhysicalDomain=network_engine_domain  SubClassName=ps_output  LeftPortType=input  RightPortType=output  PseudoPeriodic=off  Frequencies=[]  Unit=rad/s  AffineConversion=off
  PS-Simulink Converter4 : nesl_utility/PS-Simulink Converter  PhysicalDomain=network_engine_domain  SubClassName=ps_output  LeftPortType=input  RightPortType=output  PseudoPeriodic=off  Frequencies=[]  Unit=deg  AffineConversion=off
  PS-Simulink Converter5 : nesl_utility/PS-Simulink Converter  PhysicalDomain=network_engine_domain  SubClassName=ps_output  LeftPortType=input  RightPortType=output  PseudoPeriodic=off  Frequencies=[]  Unit=inherit  AffineConversion=off
  PS-Simulink Converter6 : nesl_utility/PS-Simulink Converter  PhysicalDomain=network_engine_domain  SubClassName=ps_output  LeftPortType=input  RightPortType=output  PseudoPeriodic=off  Frequencies=[]  Unit=N*m  AffineConversion=off
  actuator : Subsystem  mask{Actuator=Joint.actuator}
  motor inertia : Subsystem
  B : PMIOPort  Side=Left
  F : PMIOPort  Port=2  Side=Right
  p : Outport
  wires:
  PS-Simulink Converter5/1 -> Bus Creator1/3  "b"
  PS-Simulink Converter6/1 -> Bus Creator1/4, Abs1/1  "t"
  PS-Simulink Converter3/1 -> Bus Creator1/2  "w"
  in/1 -> actuator/1(in)
  Bus Creator1/1 -> actuator/2(fb)
  actuator/1(p) -> Bus Creator2/3  "actuator"
  Bus Creator2/1 -> p/1
  Abs1/1 -> Bus Creator2/2  "joint torque"
  PS-Simulink Converter4/1 -> Bus Creator2/1, Bus Creator1/1  "position"
  connections:
  "Hip joint "/RConn4 -- PS-Simulink Converter5/LConn1
  B/RConn1 -- motor inertia/RConn1 -- "Hip joint "/LConn1
  actuator/RConn1 -- "Hip joint "/LConn2
  "Hip joint "/RConn5 -- PS-Simulink Converter6/LConn1
  "Hip joint "/RConn2 -- PS-Simulink Converter4/LConn1
  motor inertia/LConn1 -- F/RConn1 -- "Hip joint "/RConn1
  "Hip joint "/RConn3 -- PS-Simulink Converter3/LConn1

== system quadruped_2016/robot/FL/leg/lower joint ==
  pos : Inport
  Bottom : sm_lib/Frames and Transforms/Rigid Transform  TranslationMethod=StandardAxis  TranslationStandardOffset=Leg_joint.body.length/2  TranslationLengthUnit=mm  TranslationStandardAxis=-Z  TranslationCartesianOffset=[0 0 -0.1]  TranslationROffset=0  TranslationROffsetUnits=m  TranslationZOffset=0  TranslationZOffsetUnits=m  TranslationThetaOffset=0  TranslationThetaOffsetUnits=deg  RotationMethod=StandardAxis  RotationAngleUnits=deg  RotationStandardAxis=+Y  RotationAngle=90  RotationArbitraryAxis=[0 0 1]  FollAlignAxisA=+X  BaseAlignAxisA=+Y  FollAlignAxisB=+Y  BaseAlignAxisB=+Z  RotationSequenceAxes=FollowerAxes  RotationSequence=XYX  RotationSequenceAngles=[0 0 0]  RotationSequenceAnglesUnits=deg  RotationMatrix=[1 0 0; 0 1 0; 0 0 1]
  Brick Solid : sm_lib/Body Elements/Solid  GraphicAmbientColor=[0.15 0.15 0.15 1.0]  BasedOnType=Density  BrickDimensions=Leg_joint.body.dimension  BrickDimensionUnits=mm  CenterOfMass=[0 0 0]  CenterOfMassUnits=m  GraphicDiffuseColor=Leg_joint.body.color  Density=Leg_joint.body.density  DensityUnits=kg/m^3  DoExposeReferenceFrame=on  GraphicEmissiveColor=[0.0 0.0 0.0 1.0]  ExportEntireGeometry=off  SerializedFrames=<Frames/>  MarkerShape=Sphere  MarkerSize=10  GraphicType=FromGeometry  InertiaType=CalculateFromGeometry  Mass=1  MassUnits=kg  MomentsOfInertia=[1 1 1]  MomentsOfInertiaUnits=kg*m^2  GraphicOpacity=1.0  ProductsOfInertia=[0 0 0]  ProductsOfInertiaUnits=kg*m^2  GraphicShininess=75  GraphicSpecularColor=[0.5 0.5 0.5 1.0]  GraphicVisPropType=SimpleVisualProperties  GeometryShape=Brick
  Top : sm_lib/Frames and Transforms/Rigid Transform  TranslationMethod=StandardAxis  TranslationStandardOffset=Leg_joint.body.length/2  TranslationLengthUnit=mm  TranslationStandardAxis=+Z  TranslationCartesianOffset=[0 0 0.1]  TranslationROffset=0  TranslationROffsetUnits=m  TranslationZOffset=0  TranslationZOffsetUnits=m  TranslationThetaOffset=0  TranslationThetaOffsetUnits=deg  RotationMethod=StandardAxis  RotationAngleUnits=deg  RotationStandardAxis=+Y  RotationAngle=90  RotationArbitraryAxis=[0 0 1]  FollAlignAxisA=+X  BaseAlignAxisA=+Y  FollAlignAxisB=+Y  BaseAlignAxisB=+Z  RotationSequenceAxes=FollowerAxes  RotationSequence=XYX  RotationSequenceAngles=[0 0 0]  RotationSequenceAnglesUnits=deg  RotationMatrix=[1 0 0; 0 1 0; 0 0 1]
  joint : Subsystem  mask{Joint=Leg_joint.joint}
  "B " : PMIOPort  Side=Left
  F : PMIOPort  Port=2  Side=Right
  p : Outport
  wires:
  pos/1 -> joint/1(in)
  joint/1(p) -> p/1
  connections:
  Bottom/RConn1 -- F/RConn1
  Brick Solid/RConn1 -- Bottom/LConn1 -- Top/LConn1
  "B "/RConn1 -- joint/LConn1
  joint/RConn1 -- Top/RConn1

== system quadruped_2016/robot/FL/leg/upper joint ==
  pos : Inport
  Bottom : sm_lib/Frames and Transforms/Rigid Transform  TranslationMethod=StandardAxis  TranslationStandardOffset=Leg_joint.body.length/2  TranslationLengthUnit=mm  TranslationStandardAxis=-Z  TranslationCartesianOffset=[0 0 -0.1]  TranslationROffset=0  TranslationROffsetUnits=m  TranslationZOffset=0  TranslationZOffsetUnits=m  TranslationThetaOffset=0  TranslationThetaOffsetUnits=deg  RotationMethod=StandardAxis  RotationAngleUnits=deg  RotationStandardAxis=+Y  RotationAngle=90  RotationArbitraryAxis=[0 0 1]  FollAlignAxisA=+X  BaseAlignAxisA=+Y  FollAlignAxisB=+Y  BaseAlignAxisB=+Z  RotationSequenceAxes=FollowerAxes  RotationSequence=XYX  RotationSequenceAngles=[0 0 0]  RotationSequenceAnglesUnits=deg  RotationMatrix=[1 0 0; 0 1 0; 0 0 1]
  Brick Solid : sm_lib/Body Elements/Solid  GraphicAmbientColor=[0.15 0.15 0.15 1.0]  BasedOnType=Density  BrickDimensions=Leg_joint.body.dimension  BrickDimensionUnits=mm  CenterOfMass=[0 0 0]  CenterOfMassUnits=m  GraphicDiffuseColor=Leg_joint.body.color  Density=Leg_joint.body.density  DensityUnits=kg/m^3  DoExposeReferenceFrame=on  GraphicEmissiveColor=[0.0 0.0 0.0 1.0]  ExportEntireGeometry=off  SerializedFrames=<Frames/>  MarkerShape=Sphere  MarkerSize=10  GraphicType=FromGeometry  InertiaType=CalculateFromGeometry  Mass=1  MassUnits=kg  MomentsOfInertia=[1 1 1]  MomentsOfInertiaUnits=kg*m^2  GraphicOpacity=1.0  ProductsOfInertia=[0 0 0]  ProductsOfInertiaUnits=kg*m^2  GraphicShininess=75  GraphicSpecularColor=[0.5 0.5 0.5 1.0]  GraphicVisPropType=SimpleVisualProperties  GeometryShape=Brick
  Top : sm_lib/Frames and Transforms/Rigid Transform  TranslationMethod=StandardAxis  TranslationStandardOffset=Leg_joint.body.length/2  TranslationLengthUnit=mm  TranslationStandardAxis=+Z  TranslationCartesianOffset=[0 0 0.1]  TranslationROffset=0  TranslationROffsetUnits=m  TranslationZOffset=0  TranslationZOffsetUnits=m  TranslationThetaOffset=0  TranslationThetaOffsetUnits=deg  RotationMethod=StandardAxis  RotationAngleUnits=deg  RotationStandardAxis=+Y  RotationAngle=90  RotationArbitraryAxis=[0 0 1]  FollAlignAxisA=+X  BaseAlignAxisA=+Y  FollAlignAxisB=+Y  BaseAlignAxisB=+Z  RotationSequenceAxes=FollowerAxes  RotationSequence=XYX  RotationSequenceAngles=[0 0 0]  RotationSequenceAnglesUnits=deg  RotationMatrix=[1 0 0; 0 1 0; 0 0 1]
  joint : Subsystem  mask{Joint=Leg_joint.joint}
  "B " : PMIOPort  Side=Left
  F : PMIOPort  Port=2  Side=Right
  p : Outport
  wires:
  pos/1 -> joint/1(in)
  joint/1(p) -> p/1
  connections:
  Bottom/RConn1 -- F/RConn1
  Brick Solid/RConn1 -- Bottom/LConn1 -- Top/LConn1
  "B "/RConn1 -- joint/LConn1
  joint/RConn1 -- Top/RConn1

== system quadruped_2016/robot/FR/hip/joint ==
  in : Inport
  Abs1 : Abs
  Bus Creator1 : BusCreator  Inputs=4
  Bus Creator2 : BusCreator  Inputs=3
  "Hip joint " : sm_lib/Joints/Revolute Joint  JointMode=Normal  SenseConstraintForce=off  SenseConstraintForceX=off  SenseConstraintForceY=off  SenseConstraintForceZ=off  SenseConstraintTorque=off  SenseConstraintTorqueX=off  SenseConstraintTorqueY=off  SenseConstraintTorqueZ=off  SenseTotalForce=off  SenseTotalForceX=off  SenseTotalForceY=off  SenseTotalForceZ=off  SenseTotalTorque=off  SenseTotalTorqueX=off  SenseTotalTorqueY=off  SenseTotalTorqueZ=off  CompositeWrenchDir=FollowerOnBase  CompositeWrenchFrame=BaseFrame  EquilibriumPosition=0  EquilibriumPositionUnits=rad  SpringStiffness=Joint.stiffness  SpringStiffnessUnits=N*m/deg  DampingCoefficient=Joint.damping  DampingCoefficientUnits=N*m/(deg/s)  TorqueActuationMode=InputTorque  MotionActuationMode=ComputedMotion  SensePosition=on  SenseVelocity=on  SenseAcceleration=on  SenseTorqueForce=on  SenseLowerLimitTorqueForce=off  SenseUpperLimitTorqueForce=off  LowerLimitSpecify=off  LowerLimitBound=-90  LowerLimitBoundUnits=deg  LowerLimitStiffness=1e4  LowerLimitStiffnessUnits=N*m/deg  LowerLimitDamping=10  LowerLimitDampingUnits=N*m/(deg/s)  LowerLimitTransitionRegionWidth=0.1  LowerLimitTransitionRegionWidthUnits=deg  UpperLimitSpecify=off  UpperLimitBound=90  UpperLimitBoundUnits=deg  UpperLimitStiffness=1e4  UpperLimitStiffnessUnits=N*m/deg  UpperLimitDamping=10  UpperLimitDampingUnits=N*m/(deg/s)  UpperLimitTransitionRegionWidth=0.1  UpperLimitTransitionRegionWidthUnits=deg  PositionTargetSpecify=on  PositionTargetPriority=High  PositionTargetValue=Joint.base_angle  PositionTargetValueUnits=deg  VelocityTargetSpecify=off  VelocityTargetPriority=High  VelocityTargetValue=0  VelocityTargetValueUnits=deg/s
  PS-Simulink Converter3 : nesl_utility/PS-Simulink Converter  PhysicalDomain=network_engine_domain  SubClassName=ps_output  LeftPortType=input  RightPortType=output  PseudoPeriodic=off  Frequencies=[]  Unit=rad/s  AffineConversion=off
  PS-Simulink Converter4 : nesl_utility/PS-Simulink Converter  PhysicalDomain=network_engine_domain  SubClassName=ps_output  LeftPortType=input  RightPortType=output  PseudoPeriodic=off  Frequencies=[]  Unit=deg  AffineConversion=off
  PS-Simulink Converter5 : nesl_utility/PS-Simulink Converter  PhysicalDomain=network_engine_domain  SubClassName=ps_output  LeftPortType=input  RightPortType=output  PseudoPeriodic=off  Frequencies=[]  Unit=inherit  AffineConversion=off
  PS-Simulink Converter6 : nesl_utility/PS-Simulink Converter  PhysicalDomain=network_engine_domain  SubClassName=ps_output  LeftPortType=input  RightPortType=output  PseudoPeriodic=off  Frequencies=[]  Unit=N*m  AffineConversion=off
  actuator : Subsystem  mask{Actuator=Joint.actuator}
  motor inertia : Subsystem
  B : PMIOPort  Side=Left
  F : PMIOPort  Port=2  Side=Right
  p : Outport
  wires:
  PS-Simulink Converter5/1 -> Bus Creator1/3  "b"
  PS-Simulink Converter6/1 -> Bus Creator1/4, Abs1/1  "t"
  PS-Simulink Converter3/1 -> Bus Creator1/2  "w"
  in/1 -> actuator/1(in)
  Bus Creator1/1 -> actuator/2(fb)
  actuator/1(p) -> Bus Creator2/3  "actuator"
  Bus Creator2/1 -> p/1
  Abs1/1 -> Bus Creator2/2  "joint torque"
  PS-Simulink Converter4/1 -> Bus Creator2/1, Bus Creator1/1  "position"
  connections:
  "Hip joint "/RConn4 -- PS-Simulink Converter5/LConn1
  B/RConn1 -- motor inertia/RConn1 -- "Hip joint "/LConn1
  actuator/RConn1 -- "Hip joint "/LConn2
  "Hip joint "/RConn5 -- PS-Simulink Converter6/LConn1
  "Hip joint "/RConn2 -- PS-Simulink Converter4/LConn1
  motor inertia/LConn1 -- F/RConn1 -- "Hip joint "/RConn1
  "Hip joint "/RConn3 -- PS-Simulink Converter3/LConn1
